simulink model "LQR"  (R2017a)
settings: Solver=VariableStepAuto  StartTime=0.0  StopTime=172*0.15  RelTol=1e-3
values from neighbouring files (symbols this model uses):
  Ad = inv(eye(size(A))-A.*(Ts/2))*(eye(size(A))+A.*(Ts/2))    [part2.m]    (also in part2_step_anal.m)
  Bd = inv(eye(size(A))-A.*(Ts/2))*B*Ts    [part2.m]    (also in part2_step_anal.m)
  Cd = C*inv(eye(size(A))-A.*(Ts/2))    [part2.m]    (also in part2_step_anal.m)
  Dd = D + C*inv(eye(size(A))-A.*(Ts/2))*B*(Ts/2)    [part2.m]    (also in part2_step_anal.m)
  Fmax = 180    [part2.m]    (also in part2_step_anal.m; part6_simulate.m = Fmax*gainF)
  Mmax = 10    [part2.m]    (also in part2_step_anal.m)
  Ts = 0.15    [part2.m]    (also in part2_step_anal.m)
undefined symbols (not defined in the file or in its folder): K
settings Model: Creator=zilleplus  LastModifiedBy=zilleplus

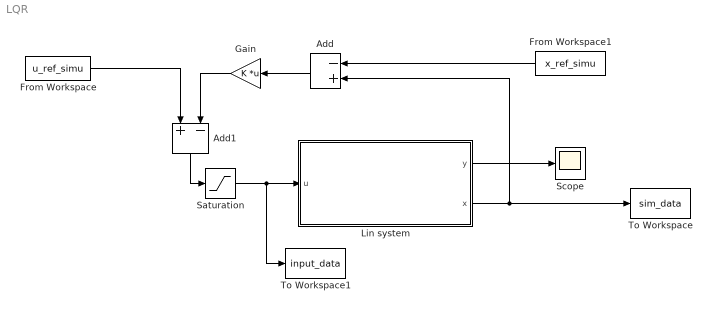
== system LQR ==
  Add : Sum  Inputs=-+
  Add1 : Sum  Inputs=+-
  From Workspace : FromWorkspace  VariableName=u_ref_simu  SampleTime=Ts
  From Workspace1 : FromWorkspace  VariableName=x_ref_simu  SampleTime=Ts
  Gain : Gain  Gain=K  Multiplication=Matrix(K*u) (u vector)
  Lin system : Subsystem
  Saturation : Saturate  UpperLimit=[Fmax;Fmax;Mmax]  LowerLimit=-[Fmax;Fmax;Mmax]
  Scope : Scope
  To Workspace : ToWorkspace  VariableName=sim_data  SaveFormat=Timeseries  SampleTime=-1
  To Workspace1 : ToWorkspace  VariableName=input_data  SaveFormat=Timeseries  SampleTime=Ts
  wires:
  Saturation/1 -> To Workspace1/1, Lin system/1(u)
  Lin system/2(x) -> Add/2, To Workspace/1
  Add/1 -> Gain/1
  From Workspace1/1 -> Add/1
  From Workspace/1 -> Add1/1
  Gain/1 -> Add1/2
  Add1/1 -> Saturation/1
  Lin system/1(y) -> Scope/1

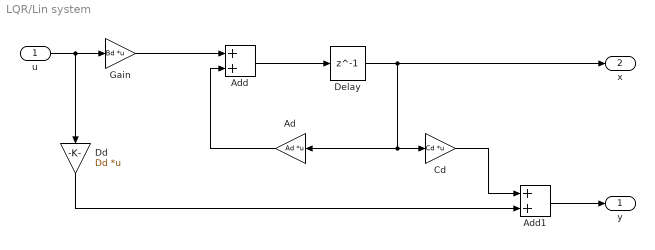
== system LQR/Lin system ==
  u : Inport
  Ad : Gain  Gain=Ad  Multiplication=Matrix(K*u) (u vector)
  Add : Sum
  Add1 : Sum
  Cd : Gain  Gain=Cd  Multiplication=Matrix(K*u) (u vector)
  Dd : Gain  Gain=Dd  Multiplication=Matrix(K*u) (u vector)
  Delay : Delay  DelayLength=1
  Gain : Gain  Gain=Bd  Multiplication=Matrix(K*u) (u vector)
  y : Outport
  x : Outport  Port=2
  wires:
  u/1 -> Dd/1, Gain/1
  Add/1 -> Delay/1
  Delay/1 -> x/1, Ad/1, Cd/1
  Ad/1 -> Add/2
  Gain/1 -> Add/1
  Cd/1 -> Add1/1
  Add1/1 -> y/1
  Dd/1 -> Add1/2
